simulink model "updowncounter_2016"  (R2016b)
settings: Solver=VariableStepAuto  StartTime=0.0  StopTime=10.0  FixedStep=1  RelTol=1e-3
settings Model: Creator=AKSHAY JP PAWAR  LastModifiedBy=AKSHAY JP PAWAR
settings DataIOCC: ReturnWorkspaceOutputs=on
settings SFSimCC: SimUseLocalCustomCode=on
settings RTWCC: RTWUseLocalCustomCode=on

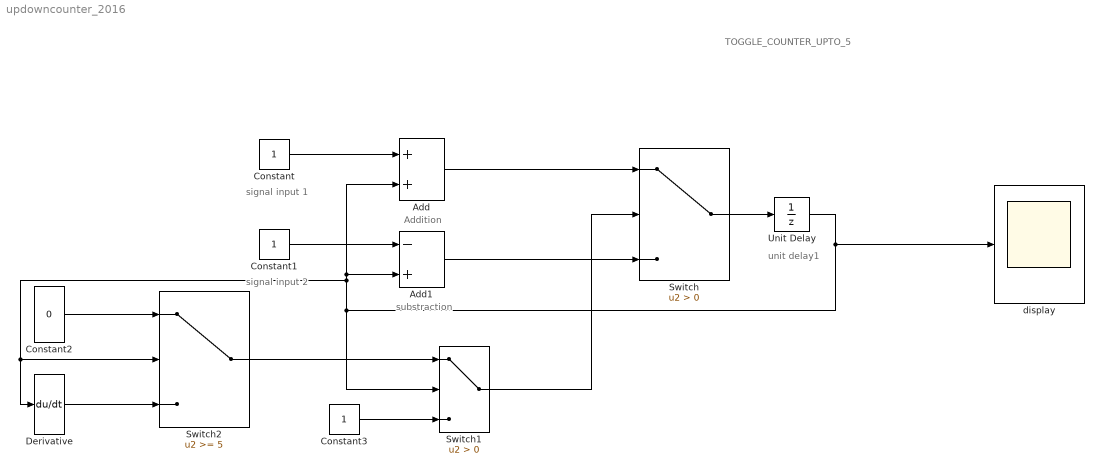
== system updowncounter_2016 ==
  note: unit delay1
  note: substraction
  note: signal input 2
  note: signal input 1
  note: TOGGLE_COUNTER_UPTO_5
  note: Addition
  Add : Sum
  Add1 : Sum  Inputs=-+
  Constant : Constant
  Constant1 : Constant
  Constant2 : Constant  Value=0
  Constant3 : Constant
  Derivative : Derivative
  Switch : Switch  Criteria=u2 > Threshold
  Switch1 : Switch  Criteria=u2 > Threshold
  Switch2 : Switch  Threshold=5
  Unit Delay : UnitDelay  SampleTime=-1  HasFrameUpgradeWarning=on
  "display " : Scope
  wires:
  Constant/1 -> Add/1
  Constant1/1 -> Add1/1
  Add/1 -> Switch/1
  Add1/1 -> Switch/3
  Switch1/1 -> Switch/2
  Switch/1 -> Unit Delay/1
  Constant2/1 -> Switch2/1
  Switch2/1 -> Switch1/1
  Constant3/1 -> Switch1/3
  Unit Delay/1 -> Switch1/2, Derivative/1, Switch2/2, Add/2, Add1/2, "display "/1
  Derivative/1 -> Switch2/3
